simulink model "pid_simulink"  (R2023a)
settings: Solver=VariableStepAuto  StartTime=0.0  StopTime=50  RelTol=1e-3
settings Model: Creator=belov  LastModifiedBy=belov

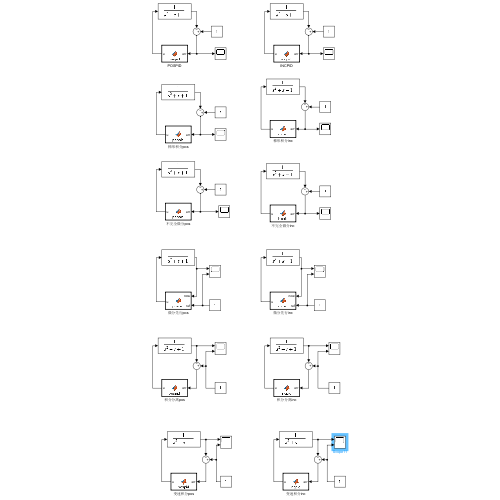
[thumbnail: Simulink's stored preview of the top-level diagram]
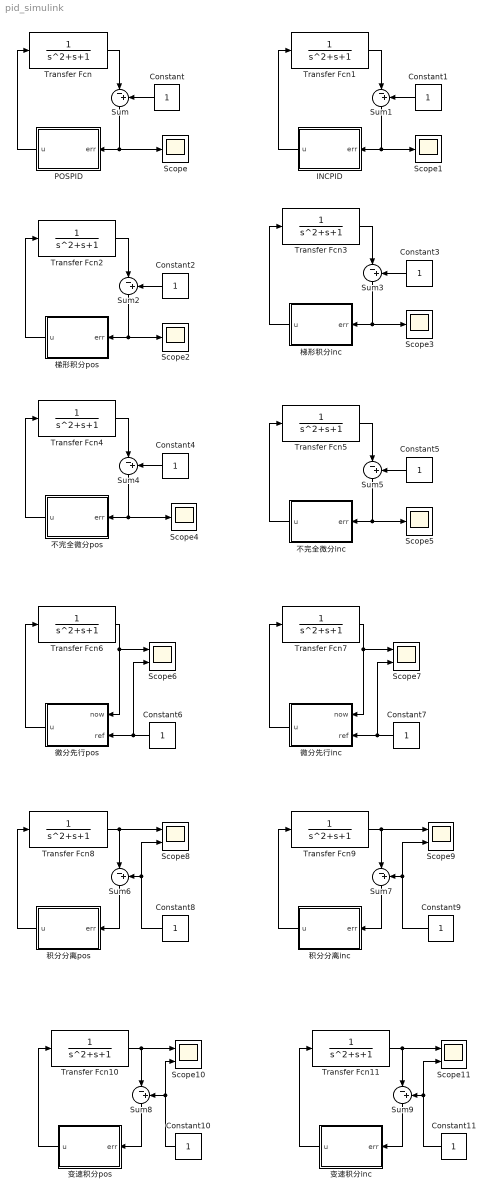
== system pid_simulink ==
  Constant{,1..11} (12 alike) : Constant  SampleTime=0.001
  INCPID : MATLAB Function  TreatAsAtomicUnit=on  SystemSampleTime=0.001
  POSPID : MATLAB Function  TreatAsAtomicUnit=on  SystemSampleTime=0.001
  Scope{,1..5} (6 alike) : Scope
  Scope{6..11} (6 alike) : Scope  NumInputPorts=2
  Sum{,1..9} (10 alike) : Sum  Inputs=|-+
  Transfer Fcn{,1..11} (12 alike) : TransferFcn  Denominator=[1 1 1]
  不完全微分inc : MATLAB Function  TreatAsAtomicUnit=on  SystemSampleTime=0.001
  不完全微分pos : MATLAB Function  TreatAsAtomicUnit=on  SystemSampleTime=0.001
  变速积分inc : MATLAB Function  TreatAsAtomicUnit=on  SystemSampleTime=0.001
  变速积分pos : MATLAB Function  TreatAsAtomicUnit=on  SystemSampleTime=0.001
  微分先行inc : MATLAB Function  TreatAsAtomicUnit=on  SystemSampleTime=0.001
  微分先行pos : MATLAB Function  TreatAsAtomicUnit=on  SystemSampleTime=0.001
  梯形积分inc : MATLAB Function  TreatAsAtomicUnit=on  SystemSampleTime=0.001
  梯形积分pos : MATLAB Function  TreatAsAtomicUnit=on  SystemSampleTime=0.001
  积分分离inc : MATLAB Function  TreatAsAtomicUnit=on  SystemSampleTime=0.001
  积分分离pos : MATLAB Function  TreatAsAtomicUnit=on  SystemSampleTime=0.001
  wires:
  POSPID/1(u) -> Transfer Fcn/1
  Transfer Fcn/1 -> Sum/1
  Sum/1 -> Scope/1, POSPID/1(err)
  Constant/1 -> Sum/2
  Constant1/1 -> Sum1/2
  Sum1/1 -> INCPID/1(err), Scope1/1
  Transfer Fcn1/1 -> Sum1/1
  INCPID/1(u) -> Transfer Fcn1/1
  Constant2/1 -> Sum2/2
  Sum2/1 -> 梯形积分pos/1(err), Scope2/1
  Transfer Fcn2/1 -> Sum2/1
  梯形积分pos/1(u) -> Transfer Fcn2/1
  梯形积分inc/1(u) -> Transfer Fcn3/1
  Transfer Fcn3/1 -> Sum3/1
  Sum3/1 -> Scope3/1, 梯形积分inc/1(err)
  Constant3/1 -> Sum3/2
  Constant4/1 -> Sum4/2
  Sum4/1 -> 不完全微分pos/1(err), Scope4/1
  Transfer Fcn4/1 -> Sum4/1
  不完全微分pos/1(u) -> Transfer Fcn4/1
  不完全微分inc/1(u) -> Transfer Fcn5/1
  Transfer Fcn5/1 -> Sum5/1
  Sum5/1 -> Scope5/1, 不完全微分inc/1(err)
  Constant5/1 -> Sum5/2
  Transfer Fcn6/1 -> 微分先行pos/1(now), Scope6/1
  Constant6/1 -> Scope6/2, 微分先行pos/2(ref)
  微分先行pos/1(u) -> Transfer Fcn6/1
  微分先行inc/1(u) -> Transfer Fcn7/1
  Constant7/1 -> 微分先行inc/2(ref), Scope7/2
  Transfer Fcn7/1 -> Scope7/1, 微分先行inc/1(now)
  Transfer Fcn8/1 -> Sum6/1, Scope8/1
  积分分离pos/1(u) -> Transfer Fcn8/1
  Transfer Fcn9/1 -> Sum7/1, Scope9/1
  积分分离inc/1(u) -> Transfer Fcn9/1
  Sum7/1 -> 积分分离inc/1(err)
  Sum6/1 -> 积分分离pos/1(err)
  Constant8/1 -> Scope8/2, Sum6/2
  Constant9/1 -> Scope9/2, Sum7/2
  Transfer Fcn10/1 -> Scope10/1, Sum8/1
  变速积分pos/1(u) -> Transfer Fcn10/1
  Transfer Fcn11/1 -> Scope11/1, Sum9/1
  变速积分inc/1(u) -> Transfer Fcn11/1
  Sum9/1 -> 变速积分inc/1(err)
  Sum8/1 -> 变速积分pos/1(err)
  Constant10/1 -> Scope10/2, Sum8/2
  Constant11/1 -> Scope11/2, Sum9/2

== matlab function pid_simulink/POSPID ==
  data: err input; u output
function u = pospid(err)

persistent accErr lasterr;
if isempty(accErr)
    accErr = 0;
end
if isempty(lasterr)
    lasterr = 0;
end

kp = 10;
ki = 0.01;
kd = 10000;
accErr = accErr + err;

u = kp * err + ki * accErr + kd * (err - lasterr);
lasterr = err;

== matlab function pid_simulink/梯形积分pos ==
  data: err input; u output
function u = pospid(err)

persistent accErr lasterr;
if isempty(accErr)
    accErr = 0;
end
if isempty(lasterr)
    lasterr = 0;
end

kp = 10;
ki = 0.01;
kd = 10000;
accErr = accErr + (err + lasterr) / 2;

u = kp * err + ki * accErr + kd * (err - lasterr);
lasterr = err;

== matlab function pid_simulink/梯形积分inc ==
  data: err input; u output
function u = incpid(err)

persistent lasterr lastlasterr usum;
if isempty(lasterr)
    lasterr = 0;
end
if isempty(lastlasterr)
    lastlasterr = 0;
end
if isempty(usum)
    usum = 0;
end


kp = 10;
ki = 0.01;
kd = 10000;

du = kp * (err - lasterr) + ki * (err + lasterr) / 2 + kd * (err - 2 * lasterr + lastlasterr);
lastlasterr = lasterr;
lasterr = err;

usum = usum + du;

u = usum;

== matlab function pid_simulink/不完全微分pos ==
  data: err input; u output
function u = pospid(err)

persistent accErr lasterr Dout;
if isempty(accErr)
    accErr = 0;
end
if isempty(lasterr)
    lasterr = 0;
end
if isempty(Dout)
    Dout = 0;
end

kp = 10;
ki = 0.01;
kd = 10000;
alpha = 0.78;
accErr = accErr + err;

Dout = alpha * Dout + (1 - alpha) * kd * (err - lasterr);

u = kp * err + ki * accErr + Dout;
lasterr = err;

== matlab function pid_simulink/不完全微分inc ==
  data: err input; u output
function u = incpid(err)

persistent lasterr lastlasterr usum deltaud;

if isempty(lasterr)
    lasterr = 0;
end
if isempty(lastlasterr)
    lastlasterr = 0;
end
if isempty(usum)
    usum = 0;
end
if isempty(deltaud)
    deltaud = 0;
end


kp = 10;
ki = 0.01;
kd = 5000;
alpha = 0.5;

deltaud = kd * (1 - alpha) * (err - 2 * lasterr + lastlasterr) + alpha * deltaud;

du = deltaud + kp * (err - lasterr) + ki * err + deltaud;

lastlasterr = lasterr;
lasterr = err;

usum = usum + du;

u = usum;

== matlab function pid_simulink/微分先行pos ==
  data: now input; u output; ref input
function u = pospid(now, ref)

persistent ud lastnow accErr;
if isempty(ud)
    ud = 0;
end
if isempty(lastnow)
    lastnow = 0;
end
if isempty(accErr)
    accErr = 0;
end

kp = 1;
ki = 0.0001;
kd = 0.003;
gamma = 0.3;

a = gamma * kd / (gamma * kd + kp);
b = (kd + kp) / (gamma * kd + kp);
c = kd / (gamma * kd + kp);

ud = ud * a + b * now + c * lastnow;

err = ref - now;
accErr = accErr + err;
u = kp * err + ki * accErr + ud;
lastnow = now;

== matlab function pid_simulink/微分先行inc ==
  data: now input; u output; ref input
function u = incpid(now, ref)

persistent deltaud lastdeltanow lasterr lastnow usum
if isempty(deltaud)
    deltaud = 0;
end
if isempty(lastdeltanow)
    lastdeltanow = 0;
end
if isempty(lasterr)
    lasterr = 0;
end
if isempty(lastnow)
    lastnow = 0;
end
if isempty(usum)
    usum = 0;
end

kp = 1;
ki = 0.0002;
kd = 0.0001;
gamma = 0.3;

deltanow = now - lastnow;
a = gamma * kd / (gamma * kd + kp);
b = (kd + kp) / (gamma * kd + kp);
c = kd / (gamma * kd + kp);

deltaud = deltaud * a + b * deltanow + c * lastdeltanow;

err = ref - now;
du = kp * (err - lasterr) + ki * err + deltaud;
usum = usum + du;
u = usum;

lastnow = now;
lastdeltanow = deltanow;
lasterr = err;

== matlab function pid_simulink/积分分离inc ==
  data: err input; u output
function u = incpid(err)

persistent lasterr lastlasterr usum;
if isempty(lasterr)
    lasterr = 0;
end
if isempty(lastlasterr)
    lastlasterr = 0;
end
if isempty(usum)
    usum = 0;
end


kp = 4;
ki = 0.001;
kd = 3000;

kiscale = 1;
if abs(err) > 0.2
    kiscale = 0;
end

du = kp * (err - lasterr) + ki * err * kiscale + kd * (err - 2 * lasterr + lastlasterr);
lastlasterr = lasterr;
lasterr = err;

usum = usum + du;

u = usum;

== matlab function pid_simulink/积分分离pos ==
  data: err input; u output
function u = pospid(err)

persistent accErr lasterr;
if isempty(accErr)
    accErr = 0;
end
if isempty(lasterr)
    lasterr = 0;
end

kp = 4;
ki = 0.001;
kd = 3000;
accErr = accErr + err;
kiscale = 1;
if abs(err) > 0.15
    kiscale = 0;
end

u = kp * err + ki * accErr * kiscale + kd * (err - lasterr);
lasterr = err;

== matlab function pid_simulink/INCPID ==
  data: err input; u output
function u = incpid(err)

persistent accErr lasterr lastlasterr usum;
if isempty(accErr)
    accErr = 0;
end
if isempty(lasterr)
    lasterr = 0;
end
if isempty(lastlasterr)
    lastlasterr = 0;
end
if isempty(usum)
    usum = 0;
end


kp = 10;
ki = 0.01;
kd = 10000;

du = kp * (err - lasterr) + ki * err + kd * (err - 2 * lasterr + lastlasterr);
lastlasterr = lasterr;
lasterr = err;

usum = usum + du;

u = usum;

== matlab function pid_simulink/变速积分inc ==
  data: err input; u output
function u = incpid(err)

persistent lasterr lastlasterr usum;

if isempty(lasterr)
    lasterr = 0;
end
if isempty(lastlasterr)
    lastlasterr = 0;
end
if isempty(usum)
    usum = 0;
end

kp = 3;
ki = 0.001;
kd = 2000;

A = 0.5;
B = 0.1;

kiscale = 0;
if abs(err) > A + B
    kiscale = 0;
elseif abs(err) > B
    kiscale = (A + B - abs(err)) / A;
else
    kiscale = 1;
end

du = kp * (err - lasterr) + ki * err * kiscale + kd * (err - 2 * lasterr + lastlasterr);
lastlasterr = lasterr;
lasterr = err;

usum = usum + du;

u = usum;

== matlab function pid_simulink/变速积分pos ==
  data: err input; u output
function u = pospid(err)

persistent accErr lasterr;
if isempty(accErr)
    accErr = 0;
end
if isempty(lasterr)
    lasterr = 0;
end

kp = 3;
ki = 0.001;
kd = 2000;


A = 0.5;
B = 0.1;

kiscale = 0;
if abs(err) > A + B
    kiscale = 0;
elseif abs(err) > B
    kiscale = (A + B - abs(err)) / A;
else
    kiscale = 1;
end

accErr = accErr + err * kiscale;

u = kp * err + ki * accErr + kd * (err - lasterr);
lasterr = err;
